simulink model "project_phase_3"  (R2026a)
settings: Solver=VariableStepAuto  StopTime=0.5
libraries: fl_lib x10, commdigbbndpm3 x4, simulink x4, nesl_utility x4, commchan3 x2, dspstat3 x2, statsLibrary x1
settings Model: Creator=DELL

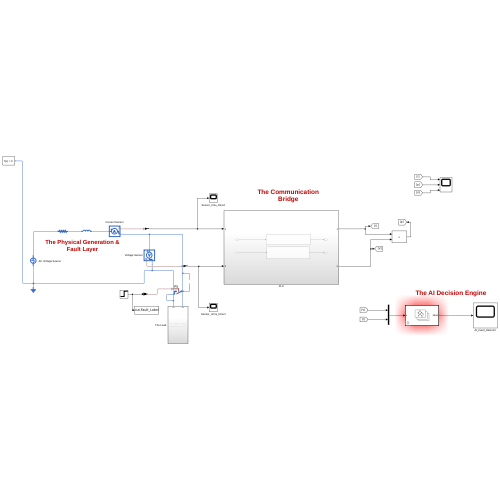
[thumbnail: Simulink's stored preview of the top-level diagram]
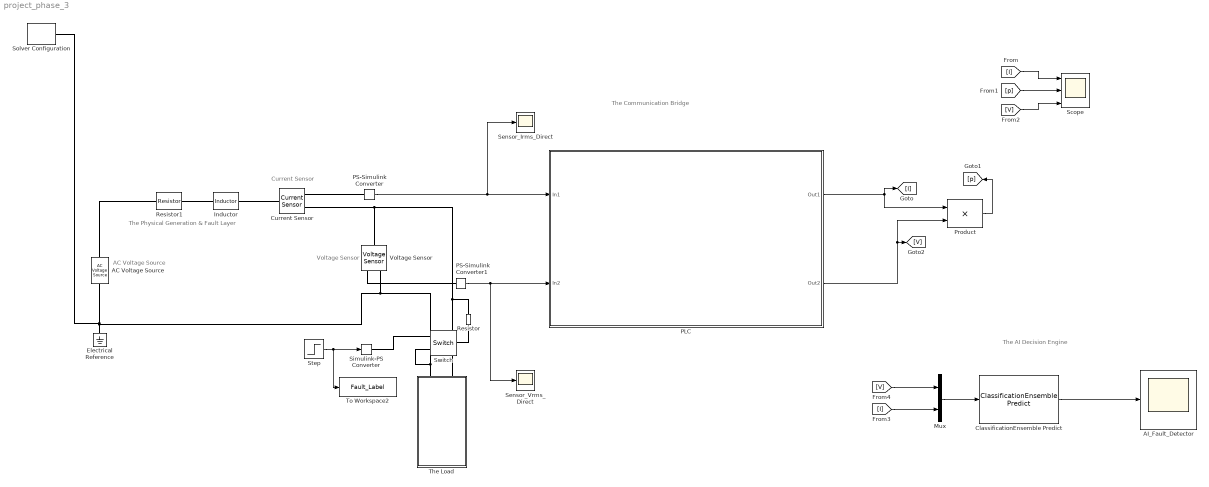
== system project_phase_3 ==
  note: The AI Decision Engine
  note: The Communication Bridge
  note: The Physical Generation & Fault Layer
  note: AC Voltage Source
  note: Voltage Sensor
  note: Current Sensor
  AC Voltage Source : fl_lib/Electrical/Electrical Sources/AC Voltage Source  amp=325 V  shift=0 deg  frequency=50 Hz
  AI_Fault_Detector : Scope
      settings: ActiveDisplayYMinimum=-0.12499999999999997  ActiveDisplayYMaximum=1.125  DataLoggingVariableName=ScopeData5
  ClassificationEnsemble Predict : statsLibrary/Classification/ClassificationEnsemble Predict  TrainedLearner=rfModel  ShowOutputScore=off  LabelDataTypeStr=Inherit: Inherit via back propagation  LabelOutMin=[]  LabelOutMax=[]  ScoreOutMin=[]  ScoreOutMax=[]  RawScoreOutMin=[]  RawScoreOutMax=[]  WeakLearnerOutMin=[]  WeakLearnerOutMax=[]  StoredEnumName=ensMdl_enumLabels
  Current Sensor : fl_lib/Electrical/Electrical Sensors/Current Sensor
  Electrical Reference : fl_lib/Electrical/Electrical Elements/Electrical Reference
  Inductor : fl_lib/Electrical/Electrical Elements/Inductor  l=1e-3 H  r=0 Ohm  g=1e-9 1/Ohm  i_specify=off  i_priority=None  i=0 A  i_nominal_specify=off  i_nominal_value=1  i_nominal_unit=A  v_specify=off  v_priority=None  v=0 V  v_nominal_specify=off  v_nominal_value=1  v_nominal_unit=V  i_L_specify=off  i_L_priority=High  i_L=0 A  i_L_nominal_specify=off  i_L_nominal_value=1  i_L_nominal_unit=A
  Mux : Mux  Inputs=2
  PLC : Subsystem
  PS-Simulink Converter : nesl_utility/PS-Simulink Converter  PhysicalDomain=network_engine_domain  SubClassName=ps_output  LeftPortType=input  RightPortType=output  PseudoPeriodic=off  Frequencies=[]  VectorFormat=inherit  Unit=inherit  AffineConversion=off
  PS-Simulink Converter1 : nesl_utility/PS-Simulink Converter  PhysicalDomain=network_engine_domain  SubClassName=ps_output  LeftPortType=input  RightPortType=output  PseudoPeriodic=off  Frequencies=[]  VectorFormat=inherit  Unit=inherit  AffineConversion=off
  Product : Product
  Resistor : fl_lib/Electrical/Electrical Elements/Resistor  R=1 Ohm  i_specify=off  i_priority=None  i=0 A  i_nominal_specify=off  i_nominal_value=1  i_nominal_unit=A  v_specify=off  v_priority=None  v=0 V  v_nominal_specify=off  v_nominal_value=1  v_nominal_unit=V
  Resistor1 : fl_lib/Electrical/Electrical Elements/Resistor  R=0.1 Ohm  i_specify=off  i_priority=None  i=0 A  i_nominal_specify=off  i_nominal_value=1  i_nominal_unit=A  v_specify=off  v_priority=None  v=0 V  v_nominal_specify=off  v_nominal_value=1  v_nominal_unit=V
  Scope : Scope  NumInputPorts=3
      settings: ActiveDisplayYMinimum=-9.7499999999999982  ActiveDisplayYMaximum=87.75
  Sensor_Irms_Direct : Scope
      settings: ActiveDisplayYMinimum=-355.1219155295297  ActiveDisplayYMaximum=355.21168816077966  DataLoggingVariableName=ScopeData2
  Sensor_Vrms_Direct : Scope
      settings: ActiveDisplayYMinimum=-405.87548681407628  ActiveDisplayYMaximum=405.8830062179137  DataLoggingVariableName=ScopeData4
  Simulink-PS Converter : nesl_utility/Simulink-PS Converter  PhysicalDomain=network_engine_domain  SubClassName=ps_input  LeftPortType=input  RightPortType=output  PseudoPeriodic=off  Frequencies=[]  NoiseDistribution=none  NoiseParameters=[]  Unit=1  AffineConversion=off  FilteringAndDerivatives=provide  SimscapeFilterOrder=1  InputFilterTimeConstant=0.001  UdotUserProvided=0
  Solver Configuration : nesl_utility/Solver Configuration  PhysicalDomain=network_engine_domain  SubClassName=solver  LeftPortType=input  RightPortType=generic  Tones=[]  Harmonics=[]  SimulateNoise=off  Profile=off  UseLocalSampling=off  EnableSwitchedLinearOptims=on  FrequencyDomain=off  UseCCode=off  RelTol=0.001  AbsTol=0.001  MinStep=1e-09  ToWorkspace=off  RevertToSquareIcSolve=off  NumHomotopyIterations=100  PhasorMode=off  PhasorModeNumHarmonics=1  ConsistencySolver=NEWTON_XTOL_AFTER_FTOL  CanonicalOrdering=CANONICAL  OptimizeIntermediates=OPTIMIZED  IndexReductionMethod=DerivativeReplacement  DoDC=off  ResidualTolerance=1e-09  ConsistencyTolSource=GLOBAL  ConsistencyAbsTol=0.001  ConsistencyRelTol=0.001  ConsistencyTolFactor=0.001  UseLocalSolver=off  LocalSolverChoice=NE_BACKWARD_EULER_ADVANCER  ResolveIndetEquations=on  FunctionEvalNumThread=1  LocalSolverSampleTime=0.001  DoFixedCost=off  MaxNonlinIter=3  MaxModeIter=2  ComputeImpulses=off  ImpulseIterations=2  LinearAlgebra=auto  LinearAlgebraNumThread=0  EquationFormulation=NE_TIME_EF  DelaysMemoryBudget=1024  AutomaticFiltering=on  FilteringTimeConstant=0.001  PartitionStorageMethod=AS_NEEDED  PartitionMemoryBudget=1024  PartitionMethod=ROBUST  MultibodyUseLocalSolver=off  MultibodyLocalSolverChoice=ODE1  MultibodyLocalSolverSampleTime=0.001
  Step : Step  Time=0.3  SampleTime=0
  Switch : fl_lib/Electrical/Electrical Elements/Switch  R_closed=0.01 Ohm  G_open=1e-8 1/Ohm  Threshold=0.5  i_specify=off  i_priority=None  i=0 A  i_nominal_specify=off  i_nominal_value=1  i_nominal_unit=A  v_specify=off  v_priority=None  v=0 V  v_nominal_specify=off  v_nominal_value=1  v_nominal_unit=V
  The Load : Subsystem
  To Workspace2 : ToWorkspace  VariableName=Fault_Label  SaveFormat=Timeseries  SampleTime=0.1
  Voltage Sensor : fl_lib/Electrical/Electrical Sensors/Voltage Sensor
  wires:
  PS-Simulink Converter/1 -> Sensor_Irms_Direct/1, PLC/1(In1)
  PS-Simulink Converter1/1 -> Sensor_Vrms_Direct/1, PLC/2(In2)
  [I] -> Scope/1
  [p] -> Scope/2
  [V] -> Scope/3
  Product/1 -> [p]
  Step/1 -> To Workspace2/1, Simulink-PS Converter/1
  PLC/1(Out1) -> [I], Product/1
  PLC/2(Out2) -> [V], Product/2
  Mux/1 -> ClassificationEnsemble Predict/1
  [V] -> Mux/1
  [I] -> Mux/2
  ClassificationEnsemble Predict/1 -> AI_Fault_Detector/1
  connections:
  Electrical Reference/LConn1 -- Switch/RConn2 -- The Load/LConn1 -- Voltage Sensor/RConn2 -- Solver Configuration/RConn1 -- AC Voltage Source/RConn1
  Inductor/LConn1 -- Resistor1/RConn1
  Resistor1/LConn1 -- AC Voltage Source/LConn1
  Current Sensor/RConn2 -- The Load/LConn2 -- Resistor/LConn1 -- Voltage Sensor/LConn1
  Inductor/RConn1 -- Current Sensor/LConn1
  Current Sensor/RConn1 -- PS-Simulink Converter/LConn1
  Voltage Sensor/RConn1 -- PS-Simulink Converter1/LConn1
  Switch/LConn1 -- Resistor/RConn1
  Simulink-PS Converter/RConn1 -- Switch/RConn1

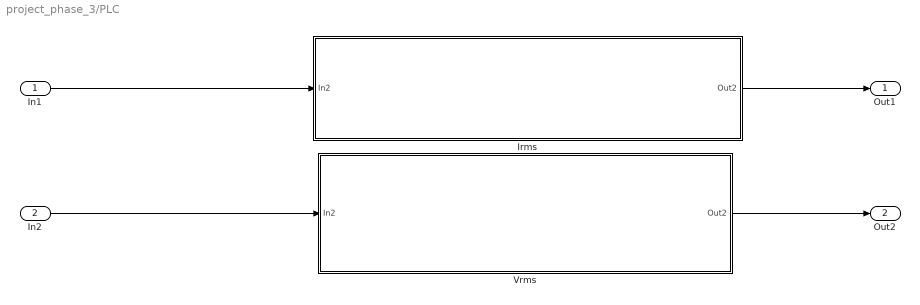
== system project_phase_3/PLC ==
  In1 : Inport
  In2 : Inport  Port=2
  Irms : Subsystem
  Vrms : Subsystem
  Out1 : Outport
  Out2 : Outport  Port=2
  wires:
  In1/1 -> Irms/1(In2)
  Irms/1(Out2) -> Out1/1
  In2/1 -> Vrms/1(In2)
  Vrms/1(Out2) -> Out2/1

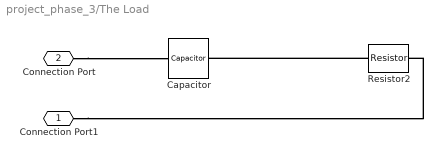
== system project_phase_3/The Load ==
  Capacitor : fl_lib/Electrical/Electrical Elements/Capacitor  c=1e-3 F  r=1e-6 Ohm  g=0 1/Ohm  i_specify=off  i_priority=None  i=0 A  i_nominal_specify=off  i_nominal_value=1  i_nominal_unit=A  v_specify=off  v_priority=None  v=0 V  v_nominal_specify=off  v_nominal_value=1  v_nominal_unit=V  vc_specify=off  vc_priority=High  vc=0 V  vc_nominal_specify=off  vc_nominal_value=1  vc_nominal_unit=V
  Resistor2 : fl_lib/Electrical/Electrical Elements/Resistor  R=100 Ohm  i_specify=off  i_priority=None  i=0 A  i_nominal_specify=off  i_nominal_value=1  i_nominal_unit=A  v_specify=off  v_priority=None  v=0 V  v_nominal_specify=off  v_nominal_value=1  v_nominal_unit=V
  Connection Port1 : PMIOPort  Side=Left
  Connection Port : PMIOPort  Port=2  Side=Left
  connections:
  Resistor2/LConn1 -- Capacitor/RConn1
  Connection Port/RConn1 -- Capacitor/LConn1
  Connection Port1/RConn1 -- Resistor2/RConn1

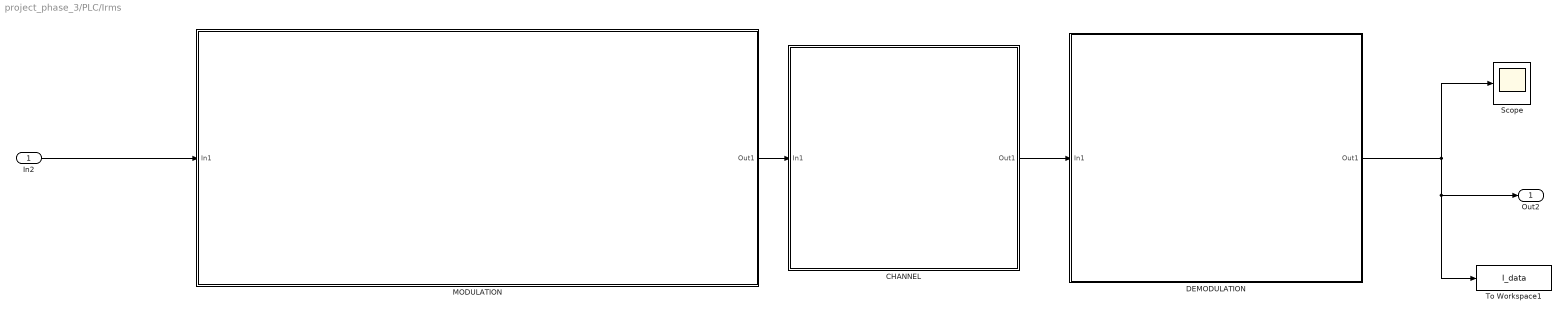
== system project_phase_3/PLC/Irms ==
  In2 : Inport
  CHANNEL : Subsystem
  DEMODULATION : Subsystem
  MODULATION : Subsystem
  Scope : Scope
      settings: ActiveDisplayYMinimum=-9.7499999999999982  ActiveDisplayYMaximum=87.75  DataLoggingVariableName=ScopeData3
  To Workspace1 : ToWorkspace  VariableName=I_data  SaveFormat=Timeseries  SampleTime=0.1
  Out2 : Outport
  wires:
  In2/1 -> MODULATION/1(In1)
  MODULATION/1(Out1) -> CHANNEL/1(In1)
  DEMODULATION/1(Out1) -> Out2/1, To Workspace1/1, Scope/1
  CHANNEL/1(Out1) -> DEMODULATION/1(In1)

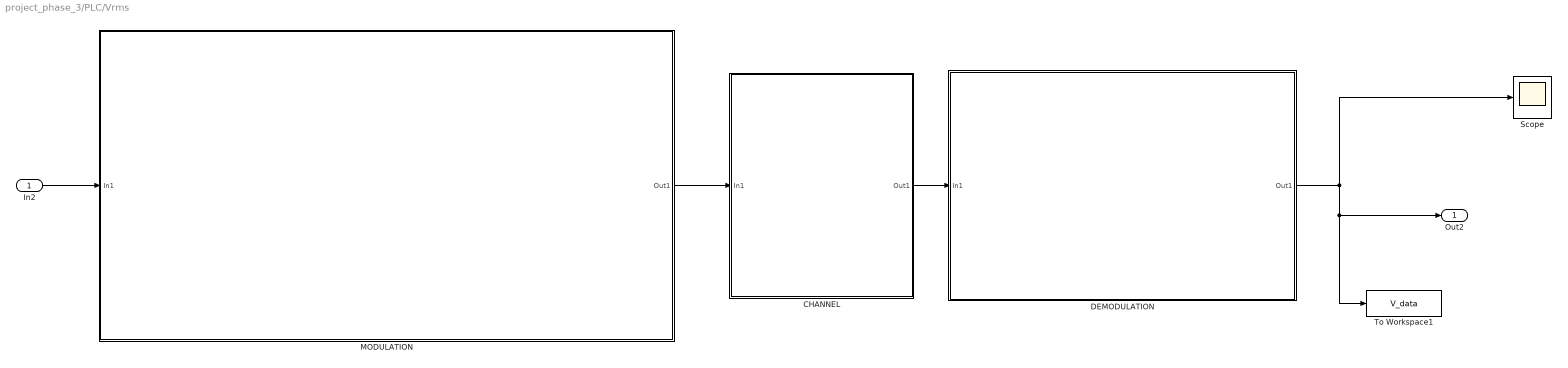
== system project_phase_3/PLC/Vrms ==
  In2 : Inport
  CHANNEL : Subsystem
  DEMODULATION : Subsystem
  MODULATION : Subsystem
  Scope : Scope
      settings: ActiveDisplayYMinimum=-2242.4999999999995  ActiveDisplayYMaximum=20182.5
  To Workspace1 : ToWorkspace  VariableName=V_data  SaveFormat=Timeseries  SampleTime=0.1
  Out2 : Outport
  wires:
  In2/1 -> MODULATION/1(In1)
  MODULATION/1(Out1) -> CHANNEL/1(In1)
  DEMODULATION/1(Out1) -> Scope/1, Out2/1, To Workspace1/1
  CHANNEL/1(Out1) -> DEMODULATION/1(In1)

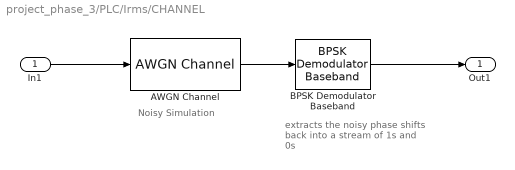
== system project_phase_3/PLC/Irms/CHANNEL ==
  note: Noisy Simulation
  note: extracts the noisy phase shifts
      | back into a stream of 1s and 0s
  In1 : Inport
  AWGN Channel : commchan3/AWGN Channel  LegacyMode=off  NoiseMethod="Signal to noise ratio  (SNR)"  noiseMode="Signal to noise ratio  (SNR)"  EbNo=10  EsNo=10  SNR=10  BitsPerSymbol=1  SignalPower=1  SpecifySymbolPeriod=off  SamplesPerSymbol=1  SymbolPeriod=1  VarianceSource=Parameter  Variance=1  RandomStream=Global stream  Seed=67  SimulateUsing=Code generation
  BPSK Demodulator Baseband : commdigbbndpm3/BPSK Demodulator Baseband  DecType=Hard decision  VarSource=Dialog  Variance=1  Ph=0  outDtype=double  derotateFactorWordLen=16  derotateFactorDataTypeStr=Inherit: Same word length as input  derotateFactorLastDataTypeStr=Inherit: Same word length as input
  Out1 : Outport
  wires:
  In1/1 -> AWGN Channel/1
  AWGN Channel/1 -> BPSK Demodulator Baseband/1
  BPSK Demodulator Baseband/1 -> Out1/1

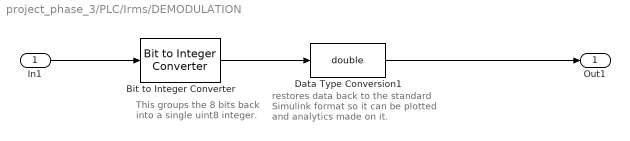
== system project_phase_3/PLC/Irms/DEMODULATION ==
  note: This groups the 8 bits back
      | into a single uint8 integer.
  note: restores data back to the standard
      | Simulink format so it can be plotted
      | and analytics made on it.
  In1 : Inport
  Bit to Integer Converter : simulink/Logic and Bit Operations/Bit to Integer Converter  nbits=8  bitOrder=MSB first  signedOutputValues=Unsigned  outDtype=uint8  outDtypeSigned=Inherit via internal rule
  Data Type Conversion1 : DataTypeConversion  OutDataTypeStr=double  SaturateOnIntegerOverflow=off  RndMeth=Floor
  Out1 : Outport
  wires:
  Bit to Integer Converter/1 -> Data Type Conversion1/1
  Data Type Conversion1/1 -> Out1/1
  In1/1 -> Bit to Integer Converter/1

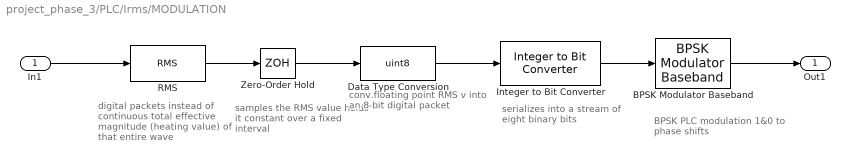
== system project_phase_3/PLC/Irms/MODULATION ==
  note: samples the RMS value
      | holds it constant over a fixed interval
  note: digital packets
      | instead of continuous
      |
      | total effective magnitude (heating value) of that entire wave
  note: conv.floating point RMS
      | v into an 8-bit digital packet
  note: serializes into a stream
      | of eight binary bits
  note: BPSK PLC modulation
      | 1&0 to phase shifts
  In1 : Inport
  BPSK Modulator Baseband : commdigbbndpm3/BPSK Modulator Baseband  Ph=0  outDtype=double  outWordLen=16  outUDDataType=sfix(16)  outFracLenMode=Best precision  outFracLen=15  outDataTypeStr=double  outLastDataTypeStr=double
  Data Type Conversion : DataTypeConversion  OutDataTypeStr=uint8  SaturateOnIntegerOverflow=off  RndMeth=Floor
  Integer to Bit Converter : simulink/Logic and Bit Operations/Integer to Bit Converter  nbits=8  signedInputValues=Unsigned  bitOrder=MSB first  outDtype=double
  RMS : dspstat3/RMS  run=off  directionMode=Each column  dimension=1  InputProcessing=Columns as channels (frame based)  reset_popup=None
  Zero-Order Hold : ZeroOrderHold  SampleTime=0.1
  Out1 : Outport
  wires:
  Zero-Order Hold/1 -> Data Type Conversion/1
  RMS/1 -> Zero-Order Hold/1
  In1/1 -> RMS/1
  Integer to Bit Converter/1 -> BPSK Modulator Baseband/1
  BPSK Modulator Baseband/1 -> Out1/1
  Data Type Conversion/1 -> Integer to Bit Converter/1

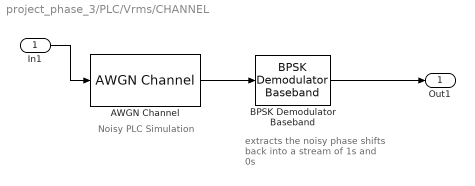
== system project_phase_3/PLC/Vrms/CHANNEL ==
  note: extracts the noisy phase shifts
      | back into a stream of 1s and 0s
  note: Noisy PLC Simulation
  In1 : Inport
  AWGN Channel : commchan3/AWGN Channel  LegacyMode=off  NoiseMethod="Signal to noise ratio  (SNR)"  noiseMode="Signal to noise ratio  (SNR)"  EbNo=10  EsNo=10  SNR=10  BitsPerSymbol=1  SignalPower=1  SpecifySymbolPeriod=off  SamplesPerSymbol=1  SymbolPeriod=1  VarianceSource=Parameter  Variance=1  RandomStream=Global stream  Seed=67  SimulateUsing=Code generation
  BPSK Demodulator Baseband : commdigbbndpm3/BPSK Demodulator Baseband  DecType=Hard decision  VarSource=Dialog  Variance=1  Ph=0  outDtype=double  derotateFactorWordLen=16  derotateFactorDataTypeStr=Inherit: Same word length as input  derotateFactorLastDataTypeStr=Inherit: Same word length as input
  Out1 : Outport
  wires:
  AWGN Channel/1 -> BPSK Demodulator Baseband/1
  In1/1 -> AWGN Channel/1
  BPSK Demodulator Baseband/1 -> Out1/1

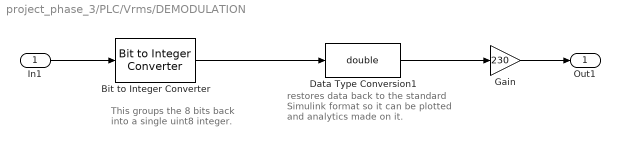
== system project_phase_3/PLC/Vrms/DEMODULATION ==
  note: restores data back to the standard
      | Simulink format so it can be plotted
      | and analytics made on it.
  note: This groups the 8 bits back
      | into a single uint8 integer.
  In1 : Inport
  Bit to Integer Converter : simulink/Logic and Bit Operations/Bit to Integer Converter  nbits=8  bitOrder=MSB first  signedOutputValues=Unsigned  outDtype=uint8  outDtypeSigned=Inherit via internal rule
  Data Type Conversion1 : DataTypeConversion  OutDataTypeStr=double  SaturateOnIntegerOverflow=off  RndMeth=Floor
  Gain : Gain  Gain=230
  Out1 : Outport
  wires:
  Data Type Conversion1/1 -> Gain/1
  Bit to Integer Converter/1 -> Data Type Conversion1/1
  In1/1 -> Bit to Integer Converter/1
  Gain/1 -> Out1/1

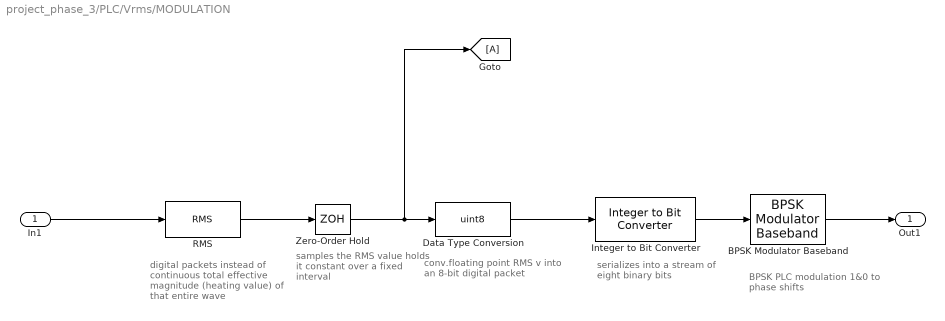
== system project_phase_3/PLC/Vrms/MODULATION ==
  note: samples the RMS value
      | holds it constant over a fixed interval
  note: BPSK PLC modulation
      | 1&0 to phase shifts
  note: serializes into a stream
      | of eight binary bits
  note: conv.floating point RMS
      | v into an 8-bit digital packet
  note: digital packets
      | instead of continuous
      |
      | total effective magnitude (heating value) of that entire wave
  In1 : Inport
  BPSK Modulator Baseband : commdigbbndpm3/BPSK Modulator Baseband  Ph=0  outDtype=double  outWordLen=16  outUDDataType=sfix(16)  outFracLenMode=Best precision  outFracLen=15  outDataTypeStr=double  outLastDataTypeStr=double
  Data Type Conversion : DataTypeConversion  OutDataTypeStr=uint8  SaturateOnIntegerOverflow=off  RndMeth=Floor
  Goto : Goto
  Integer to Bit Converter : simulink/Logic and Bit Operations/Integer to Bit Converter  nbits=8  signedInputValues=Unsigned  bitOrder=MSB first  outDtype=double
  RMS : dspstat3/RMS  run=off  directionMode=Each column  dimension=1  InputProcessing=Columns as channels (frame based)  reset_popup=None
  Zero-Order Hold : ZeroOrderHold  SampleTime=0.1
  Out1 : Outport
  wires:
  RMS/1 -> Zero-Order Hold/1
  BPSK Modulator Baseband/1 -> Out1/1
  Data Type Conversion/1 -> Integer to Bit Converter/1
  Integer to Bit Converter/1 -> BPSK Modulator Baseband/1
  Zero-Order Hold/1 -> Goto/1, Data Type Conversion/1
  In1/1 -> RMS/1
